simulink model "validation_of_wheel_component"  (R2019b)
settings: Solver=VariableStepAuto  StartTime=0.0  StopTime=10.0  RelTol=1e-3
undefined symbols (not defined in the file): m
settings Model: Creator=chiragg  LastModifiedBy=chiragg

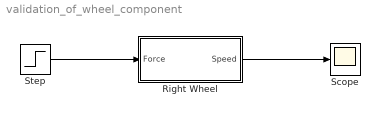
== system validation_of_wheel_component ==
  Right Wheel : Subsystem
  Scope : Scope
  Step : Step  SampleTime=0
  wires:
  Step/1 -> Right Wheel/1(Force)
  Right Wheel/1(Speed) -> Scope/1

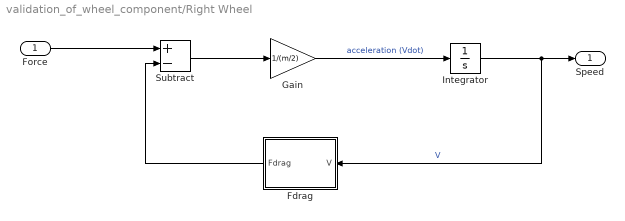
== system validation_of_wheel_component/Right Wheel ==
  Force : Inport
  Fdrag : MATLAB Function  TreatAsAtomicUnit=on
  Gain : Gain  Gain=1/(m/2)
  Integrator : Integrator
  Subtract : Sum  Inputs=+-
  Speed : Outport
  wires:
  Integrator/1 -> Fdrag/1(V), Speed/1  "V"
  Force/1 -> Subtract/1
  Fdrag/1(Fdrag) -> Subtract/2
  Subtract/1 -> Gain/1
  Gain/1 -> Integrator/1  "acceleration (Vdot)"

== matlab function validation_of_wheel_component/Right Wheel/Fdrag ==
  data: V input; Fdrag output; k_drag parameter
function Fdrag = get_fdrag(V, k_drag)

Fdrag = k_drag*V*abs(V);
